simulink model "sim_control_distance_angle"  (R2017a)
settings: Solver=VariableStepAuto  StartTime=0.0  StopTime=200  MaxStep=0.01  RelTol=1e-4  EnableMultiTasking=on
values from neighbouring files (symbols this model uses):
  Coeffd = cell2mat(den)    [control_speed.m]    (also in motor_model.m)
  Coeffn = cell2mat(num)    [control_speed.m]    (also in motor_model.m)
settings Model: Creator=hugo  LastModifiedBy=hugo
settings DataIOCC: LimitDataPoints=on  SaveOutput=off  SaveTime=off
settings OptimizationCC: ExpressionDepthLimit=2147483647  LifeSpan=1
settings DebuggingCC: UnderspecifiedInitializationDetection=Classic  MergeDetectMultiDrivingBlocksExec=none  FcnCallInpInsideContextMsg=warning  AllowSymbolicDim=off  StateNameClashWarn=warning  SFUnexpectedBacktrackingDiag=warning  SFNoUnconditionalDefaultTransitionDiag=warning  SFExecutionAtInitializationDiag=none
settings GRTTargetCC: TargetLangStandard=C89/C90 (ANSI)  GeneratePreprocessorConditionals=Disable all  CombineOutputUpdateFcns=off  GRTInterface=on

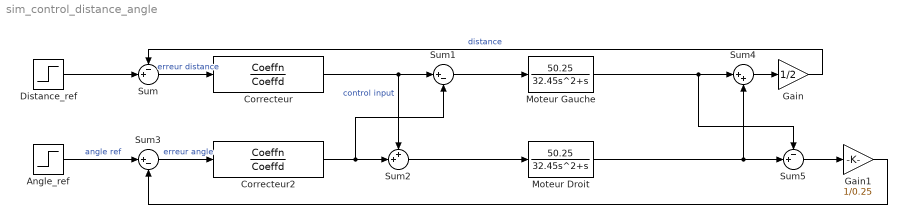
== system sim_control_distance_angle ==
  Angle_ref : Step  Time=2  After=65  SampleTime=0
  Correcteur : TransferFcn  Numerator=Coeffn  Denominator=Coeffd
  Correcteur2 : TransferFcn  Numerator=Coeffn  Denominator=Coeffd
  Distance_ref : Step  Time=6  After=50  SampleTime=0
  Gain : Gain  Gain=1/2
  Gain1 : Gain  Gain=1/0.25
  Moteur Droit : TransferFcn  Numerator=[50.25]  Denominator=[32.45 1 0]
  Moteur Gauche : TransferFcn  Numerator=[50.25]  Denominator=[32.45 1 0]
  Sum : Sum  Inputs=-+|
  Sum1 : Sum  Inputs=|+-
  Sum2 : Sum  Inputs=++|
  Sum3 : Sum  Inputs=|+-
  Sum4 : Sum  Inputs=|++
  Sum5 : Sum  Inputs=-+|
  wires:
  Sum/1 -> Correcteur/1  "erreur distance"
  Correcteur/1 -> Sum2/1, Sum1/1  "control input"
  Sum1/1 -> Moteur Gauche/1
  Sum2/1 -> Moteur Droit/1
  Sum3/1 -> Correcteur2/1  "erreur angle"
  Angle_ref/1 -> Sum3/1  "angle ref"
  Correcteur2/1 -> Sum1/2, Sum2/2
  Moteur Gauche/1 -> Sum5/1, Sum4/1
  Moteur Droit/1 -> Sum5/2, Sum4/2
  Sum4/1 -> Gain/1
  Gain/1 -> Sum/1  "distance"
  Sum5/1 -> Gain1/1
  Gain1/1 -> Sum3/2
  Distance_ref/1 -> Sum/2
